simulink model "walkingRobotOptim"  (R2019b)
settings: Solver=ode15s  StartTime=0.0  StopTime=10  EnableMultiTasking=on
PreLoadFcn:
  | robotParameters
  | 
  | % Trajectory sample time
  | tsTraj = 0.01;
  | 
  | % Simulate air drag for stability
  | world_damping = 20; % Translational damping
  | world_rot_damping = 10;  % Rotational damping
InitFcn:
  |     % Evaluate the trajectory at the start and halfway points for right and
  |     % left legs, respectively, to get initial conditions and trajectory
  |     % waypoint derivatives
  |     [q,hip_der,knee_der,ankle_der] = createSmoothTrajectory( ...
  |         hip_motion,knee_motion,ankle_motion,gait_period,[0 gait_period/2]);
  |     % Package up the initial conditions, keeping the yaw/roll joints fixed
  |     init_angs_R = [0 0 -q(1,1) -q(2,1) -q(3,1) 0];
  |     init_angs_L = [0 0 -q(1,2) -q(2,2) -q(3,2) 0];
values from neighbouring files (symbols this model uses):
  ankle_der = [0, 0.5*( diff(ankle(1:end-1)) + diff(ankle(2:end)) )/dt, 0]    [createSmoothTrajectory.m]
  ankle_motion = deg2rad([params(2*N+1:3*N), params(2*N+1)])    [simulateWalkingRobot.m]
  hip_der = [0, 0.5*( diff(hip(1:end-1)) + diff(hip(2:end)) )/dt, 0]    [createSmoothTrajectory.m]
  hip_motion = deg2rad([params(1:N), params(1)])    [simulateWalkingRobot.m]
  knee_der = [0, 0.5*( diff(knee(1:end-1)) + diff(knee(2:end)) )/dt, 0]    [createSmoothTrajectory.m]
  knee_motion = deg2rad([params(N+1:2*N), params(N+1)])    [simulateWalkingRobot.m]
  q = cubicpolytraj([hip;knee;ankle],traj_times,evalTimes,     'VelocityBoundaryCondition',[hip_der;knee_der;ankle_der])    [createSmoothTrajectory.m]
  traj_times = linspace(0,period,numPoints)    [createSmoothTrajectory.m]    (also in simulateWalkingRobot.m = linspace(0,gait_period,N+1))
undefined symbols (not defined in the file or in its folder): gait_period
libraries: simulink x2, robotcorelib x2, walkingRobotUtils x2
settings Model: Creator=bkim  LastModifiedBy=scastro
settings DataIOCC: ReturnWorkspaceOutputs=off  OutputSaveName=simout  OutputTimes=0:0.01:10
settings OptimizationCC: LifeSpan=inf
settings DebuggingCC: AllowSymbolicDim=off  PregeneratedLibrarySubsystemCodeDiagnostic=none  SFUnexpectedBacktrackingDiag=warning  SFNoUnconditionalDefaultTransitionDiag=warning  SFExecutionAtInitializationDiag=none  UnitsInconsistencyMsg=none  ArithmeticOperatorsInVariantConditions=warning
settings SFSimCC: SimUseLocalCustomCode=off  CustomCodeUndefinedFunction=UseInterfaceOnly
settings RTWCC: RTWUseLocalCustomCode=off
settings CodeAppCC: StateflowObjectComments=on
settings GRTTargetCC: TargetLangStandard=C89/C90 (ANSI)  GeneratePreprocessorConditionals=Disable all
settings ConfigComp: CovMetricSettings=dw  CovHtmlReporting=on  CovSaveCumulativeToWorkspaceVar=on  CovSaveSingleToWorkspaceVar=on  CovExternalEMLEnable=off  CovSFcnEnable=off
settings SimscapeCC: SimscapeNormalizeSystem=off  SimscapeLogOpenViewer=on  SimscapeLogLimitData=off  SimscapeLogDataHistory=10000
settings ConfigurationSet: Description=SimMechanics 2G
settings DiagnosticsConfigSet: SimMechanicsRigidlyBoundBlock=none
settings ExplorerConfigSet: InternalSimMechanicsExplorerSettings="<ExplorerConfiguration><canonicalview>default</canonicalview><AnimationSetting><BasePlaybackSpeed>1.0</BasePlaybackSpeed><PlaybackSpeedFactor>1.0</PlaybackSpeedFactor></AnimationSetting><TilePanel><TileInfo><Tiles Columns=\"1\" Count=\"1\" Rows=\"1\"><Column Weight=\"1\"/><Row Weight=\"1\"/><Tile Height=\"1\" Width=\"1\" X=\"0\" Y=\"0\"/></Tiles></TileInfo><SceneInfo><SceneViewer><BGColor><R>0.60000002384185791</R><G>0.60000002384185791</G><B>0.60000002384185791</B></BGColor><Camera><DoPerspective>off</DoPerspective><Position><X>-6.96629667239135308</X><Y>24.6054722866086557</Y><Z>5.12968018743748999</Z></Position><Center><X>2.4732135105562727</X><Y>-3.90012739093662164</Y><Z>-2.29509835736230228</Z></Center><Up><X>0.317576681516579584</X><Y>-0.139145800878009762</Y><Z>0.937967748621952424</Z></Up><ViewLimDist>1</ViewLimDist><YLim>3.00115752214017162</YLim><XLim>3.84407522125978751</XLim></Camera></SceneViewer></SceneInfo></TilePanel><MechEditorPanel><Cameras/><GfxPanelCameraMap/><VideoCreator><PlaybackSpeedRatio>1.0</PlaybackSpeedRatio><FrameRate>30</FrameRate><VideoFormat>Motion JPEG AVI</VideoFormat><FrameSize>auto</FrameSize></VideoCreator></MechEditorPanel></ExplorerConfiguration>"

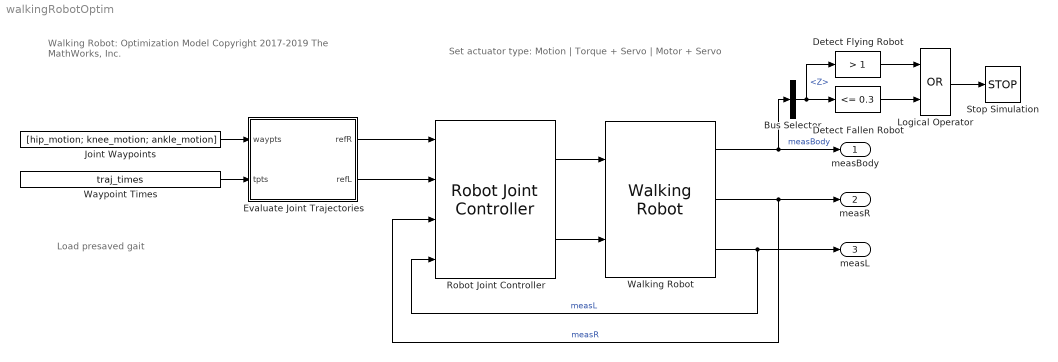
== system walkingRobotOptim ==
  note: Load presaved gait
  note: Walking Robot: Optimization Model
      |
      | Copyright 2017-2019 The MathWorks, Inc.
  note: Set actuator type:
      | Motion | Torque + Servo | Motor + Servo
  Bus Selector : BusSelector  OutputSignals=Z
  Detect Fallen Robot : simulink/Logic and Bit Operations/Compare To Constant  relop=<=  const=0.3  OutDataTypeStr=boolean
  Detect Flying Robot : simulink/Logic and Bit Operations/Compare To Constant  relop=>  const=1  OutDataTypeStr=boolean
  Evaluate Joint Trajectories : Subsystem
  Joint Waypoints : Constant  Value=[hip_motion; knee_motion; ankle_motion]
  Logical Operator : Logic  Operator=OR  AllPortsSameDT=off  OutDataTypeStr=boolean
  Robot Joint Controller : walkingRobotUtils/Robot Joint Controller  SystemSampleTime=-1  Latency=0  AutoFrameSizeCalculation=off
  Stop Simulation : Stop
  Walking Robot : walkingRobotUtils/Walking Robot  SystemSampleTime=-1  Latency=0  AutoFrameSizeCalculation=off
  Waypoint Times : Constant  Value=traj_times
  measBody : Outport  VectorParamsAs1DForOutWhenUnconnected=off
  measR : Outport  Port=2  VectorParamsAs1DForOutWhenUnconnected=off
  measL : Outport  Port=3  VectorParamsAs1DForOutWhenUnconnected=off
  wires:
  Walking Robot/3 -> Robot Joint Controller/4, measL/1  "measL"
  Walking Robot/2 -> Robot Joint Controller/3, measR/1  "measR"
  Robot Joint Controller/1 -> Walking Robot/1
  Robot Joint Controller/2 -> Walking Robot/2
  Evaluate Joint Trajectories/1(refR) -> Robot Joint Controller/1
  Evaluate Joint Trajectories/2(refL) -> Robot Joint Controller/2
  Walking Robot/1 -> Bus Selector/1, measBody/1  "measBody"
  Bus Selector/1 -> Detect Fallen Robot/1, Detect Flying Robot/1  "<Z>"
  Detect Fallen Robot/1 -> Logical Operator/2
  Joint Waypoints/1 -> Evaluate Joint Trajectories/1(waypts)
  Waypoint Times/1 -> Evaluate Joint Trajectories/2(tpts)
  Logical Operator/1 -> Stop Simulation/1
  Detect Flying Robot/1 -> Logical Operator/1

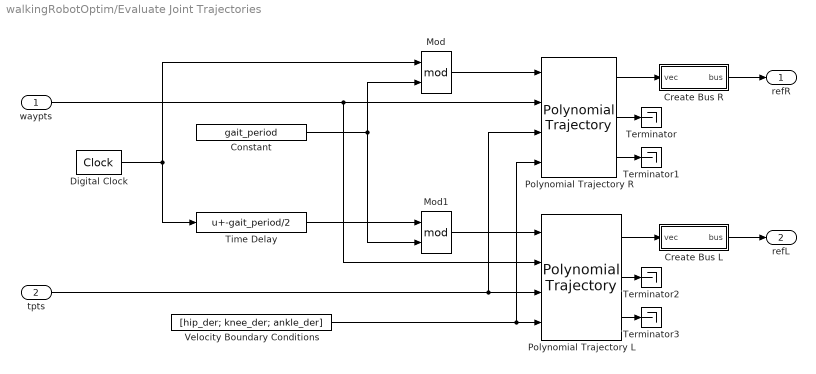
== system walkingRobotOptim/Evaluate Joint Trajectories ==
  waypts : Inport
  tpts : Inport  Port=2
  Constant : Constant  Value=gait_period
  Create Bus L : Subsystem
  Create Bus R : Subsystem
  Digital Clock : DigitalClock  SampleTime=tsTraj
  Mod : Math  Operator=mod  SignedPower=off  SaturateOnIntegerOverflow=on
  Mod1 : Math  Operator=mod  SignedPower=off  SaturateOnIntegerOverflow=on
  Polynomial Trajectory L : robotcorelib/Polynomial Trajectory  WaypointSource=External  Waypoints=[ 0, 2, 1, 5, 0; -1, 3, 1, 4, 4 ]  TimePoints=time  TimeInterval=[ 1, 4 ]  Method=Cubic Polynomial  ParameterSource=External  VelocityBoundaryCondition=[hip_der; knee_der; ankle_der]  AccelerationBoundaryCondition=zeros( 2, 5 )  SimulateUsing=Interpreted execution
      settings: SourceProductName=Robotics System Toolbox  SourceProductBaseCode=RO
  Polynomial Trajectory R : robotcorelib/Polynomial Trajectory  WaypointSource=External  Waypoints=[ 0, 2, 1, 5, 0; -1, 3, 1, 4, 4 ]  TimePoints=time  TimeInterval=[ 1, 4 ]  Method=Cubic Polynomial  ParameterSource=External  VelocityBoundaryCondition=[hip_der; knee_der; ankle_der]  AccelerationBoundaryCondition=zeros( 2, 5 )  SimulateUsing=Interpreted execution
      settings: SourceProductName=Robotics System Toolbox  SourceProductBaseCode=RO
  Terminator{,1..3} (4 alike) : Terminator
  Time Delay : Bias  Bias=-gait_period/2
  Velocity Boundary Conditions : Constant  Value=[hip_der; knee_der; ankle_der]
  refR : Outport
  refL : Outport  Port=2
  wires:
  Polynomial Trajectory R/1 -> Create Bus R/1(vec)
  Create Bus L/1(bus) -> refL/1
  Create Bus R/1(bus) -> refR/1
  Polynomial Trajectory L/1 -> Create Bus L/1(vec)
  Mod1/1 -> Polynomial Trajectory L/1
  tpts/1 -> Polynomial Trajectory R/3, Polynomial Trajectory L/3
  Time Delay/1 -> Mod1/1
  Polynomial Trajectory L/3 -> Terminator3/1
  Polynomial Trajectory R/2 -> Terminator/1
  Polynomial Trajectory R/3 -> Terminator1/1
  Polynomial Trajectory L/2 -> Terminator2/1
  Constant/1 -> Mod/2, Mod1/2
  waypts/1 -> Polynomial Trajectory R/2, Polynomial Trajectory L/2
  Mod/1 -> Polynomial Trajectory R/1
  Digital Clock/1 -> Time Delay/1, Mod/1
  Velocity Boundary Conditions/1 -> Polynomial Trajectory R/4, Polynomial Trajectory L/4

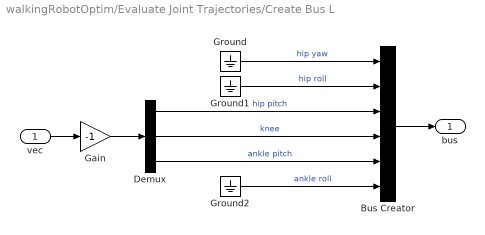
== system walkingRobotOptim/Evaluate Joint Trajectories/Create Bus L ==
  vec : Inport
  Bus Creator : BusCreator  Inputs=6
  Demux : Demux  Outputs=3
  Gain : Gain  Gain=-1
  Ground : Ground
  Ground1 : Ground
  Ground2 : Ground
  bus : Outport  VectorParamsAs1DForOutWhenUnconnected=off
  wires:
  Demux/1 -> Bus Creator/3  "hip pitch"
  Ground/1 -> Bus Creator/1  "hip yaw"
  Demux/3 -> Bus Creator/5  "ankle pitch"
  Ground1/1 -> Bus Creator/2  "hip roll"
  Demux/2 -> Bus Creator/4  "knee"
  Ground2/1 -> Bus Creator/6  "ankle roll"
  vec/1 -> Gain/1
  Bus Creator/1 -> bus/1
  Gain/1 -> Demux/1

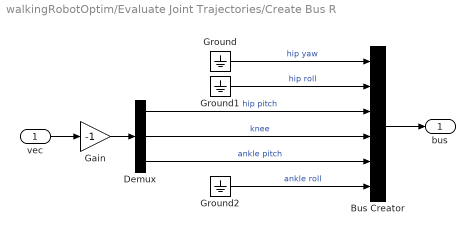
== system walkingRobotOptim/Evaluate Joint Trajectories/Create Bus R ==
  vec : Inport
  Bus Creator : BusCreator  Inputs=6
  Demux : Demux  Outputs=3
  Gain : Gain  Gain=-1
  Ground : Ground
  Ground1 : Ground
  Ground2 : Ground
  bus : Outport  VectorParamsAs1DForOutWhenUnconnected=off
  wires:
  Bus Creator/1 -> bus/1
  vec/1 -> Gain/1
  Ground2/1 -> Bus Creator/6  "ankle roll"
  Demux/2 -> Bus Creator/4  "knee"
  Ground1/1 -> Bus Creator/2  "hip roll"
  Demux/3 -> Bus Creator/5  "ankle pitch"
  Ground/1 -> Bus Creator/1  "hip yaw"
  Demux/1 -> Bus Creator/3  "hip pitch"
  Gain/1 -> Demux/1
